simulink model "Vehicle_M2018b"  (R2018a)
settings: Solver=VariableStepAuto  StartTime=0.0  StopTime=5  MaxStep=0.01  RelTol=1e-3
settings Model: Creator=Nitzsche  LastModifiedBy=Ossmann

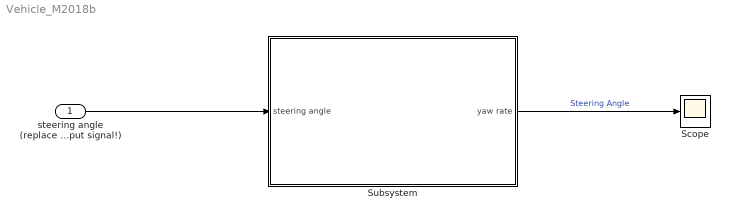
== system Vehicle_M2018b ==
  steering angle (replace with your input signal!) : Inport
  Scope : Scope
  Subsystem : Subsystem  mask{EinAus=<empty>}
      mask prompts: EinAus "BMW1"
      mask TypeOptions EinAus: <empty>
      mask Display: image(imread('car.bmp'))
  wires:
  Subsystem/1(yaw rate) -> Scope/1  "Steering Angle"
  steering angle (replace with your input signal!)/1 -> Subsystem/1(steering angle)

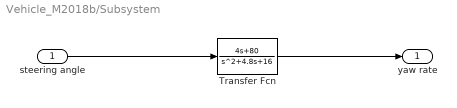
== system Vehicle_M2018b/Subsystem ==
  steering angle : Inport
  Transfer Fcn : TransferFcn  Numerator=[4 80]  Denominator=[1 4.8 16]
  yaw rate : Outport
  wires:
  steering angle/1 -> Transfer Fcn/1
  Transfer Fcn/1 -> yaw rate/1
